simulink model "converter_simulink"  (R2024b)
settings: Solver=FixedStepDiscrete  StartTime=0.0  StopTime=10.0  FixedStep=1  RelTol=1e-3
settings Model: Creator=samue  LastModifiedBy=samue

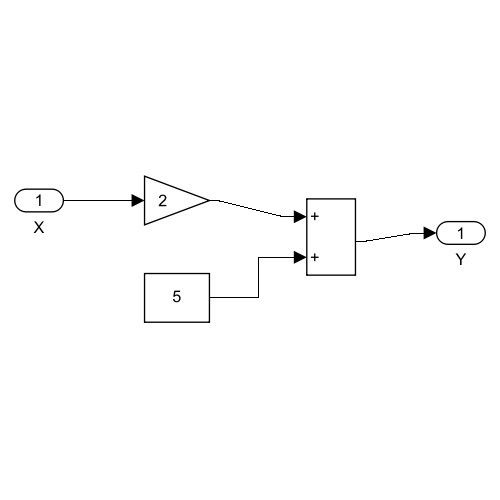
[thumbnail: Simulink's stored preview of the top-level diagram]
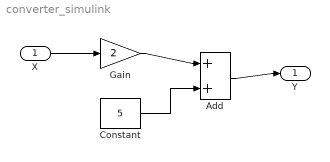
== system converter_simulink ==
  X : Inport  OutDataTypeStr=uint8  SampleTime=1
  Add : Sum
  Constant : Constant  Value=5  OutDataTypeStr=uint8
  Gain : Gain  Gain=2  OutDataTypeStr=Inherit: Same as input
  Y : Outport
  wires:
  X/1 -> Gain/1
  Gain/1 -> Add/1
  Constant/1 -> Add/2
  Add/1 -> Y/1
